simulink model "project"  (R2020a)
settings: Solver=ode15s  StartTime=0.0  StopTime=0.1  RelTol=1e-3
settings Model: Creator=M VEMAN SAI PRABHATH  LastModifiedBy=M VEMAN SAI PRABHATH
settings SolverCC: ZeroCrossAlgorithm=Adaptive
settings DebuggingCC: IgnoredZcDiagnostic=none
settings SFSimCC: CustomCodeUndefinedFunction=UseInterfaceOnly

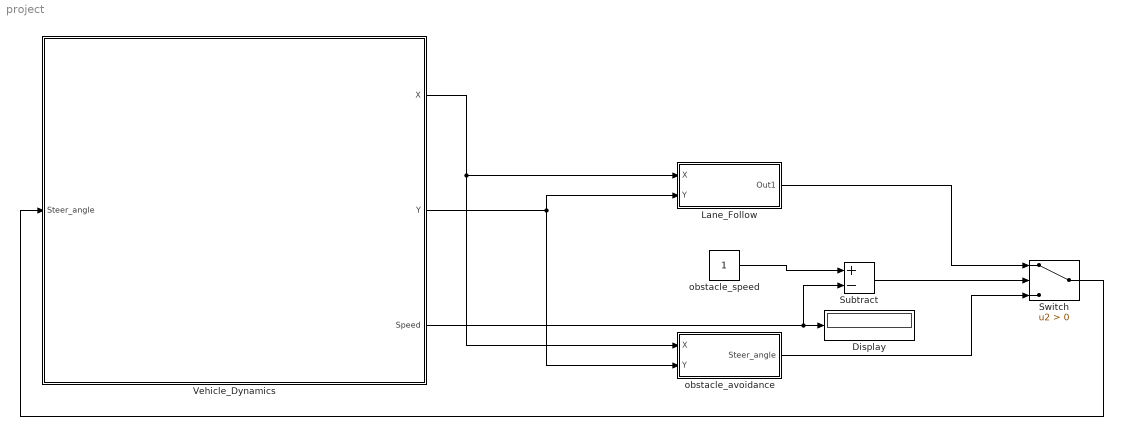
== system project ==
  Display : Display
  Lane_Follow : Subsystem
  Subtract : Sum  Inputs=+-
  Switch : Switch  Criteria=u2 > Threshold
  Vehicle_Dynamics : Subsystem
  obstacle_avoidance : Subsystem
  obstacle_speed : Constant
  wires:
  Vehicle_Dynamics/1(X) -> obstacle_avoidance/1(X), Lane_Follow/1(X)
  Vehicle_Dynamics/2(Y) -> obstacle_avoidance/2(Y), Lane_Follow/2(Y)
  Vehicle_Dynamics/3(Speed) -> Subtract/2, Display/1
  obstacle_speed/1 -> Subtract/1
  Subtract/1 -> Switch/2
  Switch/1 -> Vehicle_Dynamics/1(Steer_angle)
  Lane_Follow/1(Out1) -> Switch/1
  obstacle_avoidance/1(Steer_angle) -> Switch/3

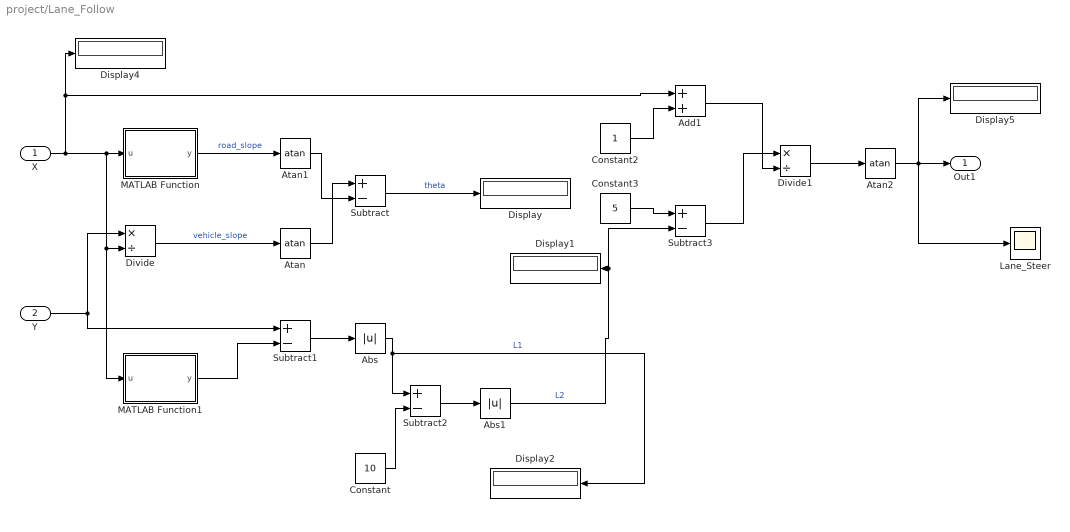
== system project/Lane_Follow ==
  X : Inport
  Y : Inport  Port=2
  Abs : Abs
  Abs1 : Abs
  Add1 : Sum
  Atan : Trigonometry  Operator=atan
  Atan1 : Trigonometry  Operator=atan
  Atan2 : Trigonometry  Operator=atan
  Constant : Constant  Value=10
  Constant2 : Constant
  Constant3 : Constant  Value=5
  Display{,1..2,4..5} (5 alike) : Display
  Divide : Product  Inputs=*/
  Divide1 : Product  Inputs=*/
  Lane_Steer : Scope
  MATLAB Function : MATLAB Function  TreatAsAtomicUnit=on
  MATLAB Function1 : MATLAB Function  TreatAsAtomicUnit=on
  Subtract{,1..3} (4 alike) : Sum  Inputs=+-
  Out1 : Outport
  wires:
  Y/1 -> Divide/1, Subtract1/1
  X/1 -> Add1/1, Display4/1, MATLAB Function/1(u), MATLAB Function1/1(u), Divide/2
  Divide/1 -> Atan/1  "vehicle_slope"
  MATLAB Function/1(y) -> Atan1/1  "road_slope"
  Atan/1 -> Subtract/1
  Atan1/1 -> Subtract/2
  Subtract/1 -> Display/1  "theta"
  MATLAB Function1/1(y) -> Subtract1/2
  Subtract1/1 -> Abs/1
  Abs/1 -> Display2/1, Subtract2/1  "L1"
  Constant/1 -> Subtract2/2
  Subtract2/1 -> Abs1/1
  Abs1/1 -> Subtract3/2, Display1/1  "L2"
  Constant2/1 -> Add1/2
  Constant3/1 -> Subtract3/1
  Subtract3/1 -> Divide1/1
  Add1/1 -> Divide1/2
  Divide1/1 -> Atan2/1
  Atan2/1 -> Lane_Steer/1, Display5/1, Out1/1

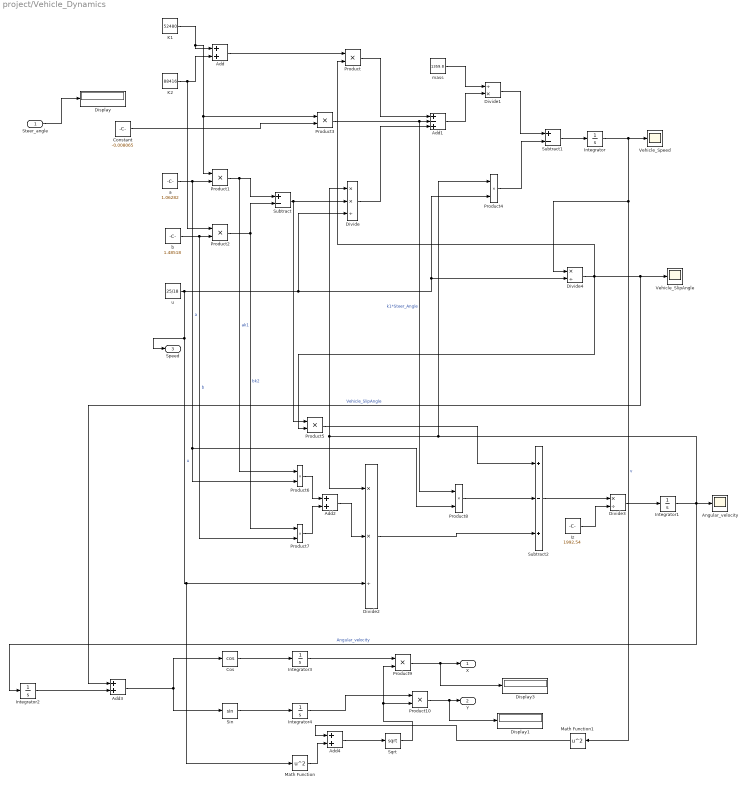
== system project/Vehicle_Dynamics ==
  Steer_angle : Inport
  Add{,2..4} (4 alike) : Sum
  Add1 : Sum  Inputs=+-+
  Angular_velocity : Scope
  Constant : Constant  Value=-0.008065
  Cos : Trigonometry  Operator=cos
  Display : Display
  Display1 : Display
  Display3 : Display
  Divide : Product  Inputs=**/
  Divide1 : Product  Inputs=/*
  Divide2 : Product  Inputs=**/
  Divide3 : Product  Inputs=*/
  Divide4 : Product  Inputs=*/
  Integrator : Integrator  ZeroCross=off
  Integrator{1..4} (4 alike) : Integrator
  Iz : Constant  Value=1992.54
  K1 : Constant  Value=52480
  K2 : Constant  Value=88416
  Math Function : Math  Operator=square  SignedPower=on  SaturateOnIntegerOverflow=on
  Math Function1 : Math  Operator=square  SignedPower=on  SaturateOnIntegerOverflow=on
  Product{,1..10} (11 alike) : Product
  Sin : Trigonometry
  Sqrt : Sqrt  SaturateOnIntegerOverflow=on
  Subtract : Sum  Inputs=+-
  Subtract1 : Sum  Inputs=+-
  Subtract2 : Sum  Inputs=+-+
  Vehicle_SlipAngle : Scope
  Vehicle_Speed : Scope
  a : Constant  Value=1.06282
  b : Constant  Value=1.48518
  mass : Constant  Value=1359.8
  u : Constant  Value=25/18
  X : Outport  VectorParamsAs1DForOutWhenUnconnected=off
  Y : Outport  Port=2  VectorParamsAs1DForOutWhenUnconnected=off
  Speed : Outport  Port=3
  wires:
  u/1 -> Speed/1, Math Function/1, Divide2/3, Divide4/2, Product4/2, Divide/3  "u"
  mass/1 -> Divide1/1
  Subtract/1 -> Product5/1, Divide/2
  Add/1 -> Product/1
  K2/1 -> Product2/1, Add/2
  Product2/1 -> Product7/1, Subtract/2  "bk2"
  K1/1 -> Product3/1, Product1/1, Add/1
  b/1 -> Product7/2, Product2/2  "b"
  Product1/1 -> Product6/1, Subtract/1  "ak1"
  Add1/1 -> Divide1/2
  Divide4/1 -> Product5/2, Add3/1, Vehicle_SlipAngle/1, Product/2  "Vehicle_SlipAngle"
  Subtract1/1 -> Integrator/1
  Divide1/1 -> Subtract1/1
  Product4/1 -> Subtract1/2
  Divide/1 -> Add1/3
  Product/1 -> Add1/1
  Product3/1 -> Product8/1, Add1/2  "k1*Steer_Angle"
  a/1 -> Product8/2, Product6/2, Product1/2  "a"
  Product6/1 -> Add2/1
  Product7/1 -> Add2/2
  Add2/1 -> Divide2/2
  Integrator1/1 -> Integrator2/1, Product4/1, Divide2/1, Divide/1, Angular_velocity/1  "Angular_velocity"
  Divide2/1 -> Subtract2/3
  Product5/1 -> Subtract2/1
  Product8/1 -> Subtract2/2
  Subtract2/1 -> Divide3/1
  Iz/1 -> Divide3/2
  Divide3/1 -> Integrator1/1
  Integrator/1 -> Math Function1/1, Divide4/1, Vehicle_Speed/1  "v"
  Integrator2/1 -> Add3/2
  Add3/1 -> Sin/1, Cos/1
  Cos/1 -> Integrator3/1
  Sin/1 -> Integrator4/1
  Math Function1/1 -> Add4/1
  Math Function/1 -> Add4/2
  Add4/1 -> Sqrt/1
  Sqrt/1 -> Product10/2, Product9/2
  Integrator3/1 -> Product9/1
  Integrator4/1 -> Product10/1
  Product9/1 -> Display3/1, X/1
  Product10/1 -> Display1/1, Y/1
  Constant/1 -> Product3/2
  Steer_angle/1 -> Display/1

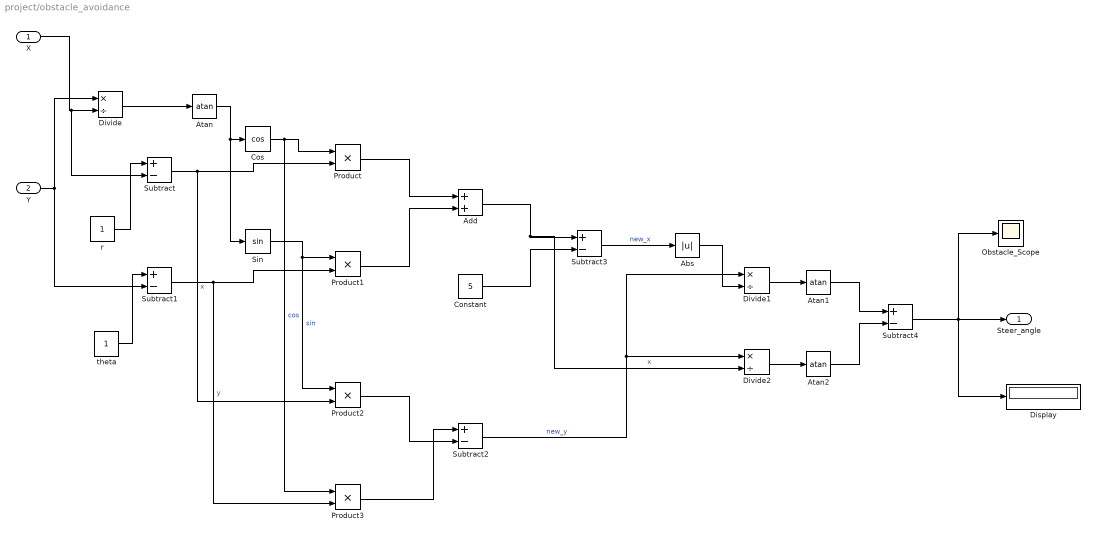
== system project/obstacle_avoidance ==
  X : Inport
  Y : Inport  Port=2
  Abs : Abs
  Add : Sum
  Atan : Trigonometry  Operator=atan
  Atan1 : Trigonometry  Operator=atan
  Atan2 : Trigonometry  Operator=atan
  Constant : Constant  Value=5
  Cos : Trigonometry  Operator=cos
  Display : Display
  Divide : Product  Inputs=*/
  Divide1 : Product  Inputs=*/
  Divide2 : Product  Inputs=*/
  Obstacle_Scope : Scope
  Product{,1..3} (4 alike) : Product
  Sin : Trigonometry
  Subtract{,1..4} (5 alike) : Sum  Inputs=+-
  r : Constant
  theta : Constant
  Steer_angle : Outport  VectorParamsAs1DForOutWhenUnconnected=off
  wires:
  X/1 -> Subtract/2, Divide/2
  Y/1 -> Subtract1/2, Divide/1
  Divide/1 -> Atan/1
  r/1 -> Subtract/1
  Atan/1 -> Sin/1, Cos/1
  Cos/1 -> Product3/1, Product/1  "cos"
  Subtract/1 -> Product2/2, Product/2  "x"
  theta/1 -> Subtract1/1
  Subtract1/1 -> Product3/2, Product1/2  "y"
  Sin/1 -> Product2/1, Product1/1  "sin"
  Product/1 -> Add/1
  Product1/1 -> Add/2
  Product2/1 -> Subtract2/2
  Product3/1 -> Subtract2/1
  Constant/1 -> Subtract3/2
  Add/1 -> Divide2/2, Subtract3/1  "x"
  Subtract3/1 -> Abs/1  "new_x"
  Abs/1 -> Divide1/2
  Subtract2/1 -> Divide1/1, Divide2/1  "new_y"
  Divide1/1 -> Atan1/1
  Divide2/1 -> Atan2/1
  Atan1/1 -> Subtract4/1
  Atan2/1 -> Subtract4/2
  Subtract4/1 -> Obstacle_Scope/1, Display/1, Steer_angle/1

== matlab function project/Lane_Follow/MATLAB Function ==
  data: u input; y output
function y = fcn(u)

y = (2*u) - 5;

== matlab function project/Lane_Follow/MATLAB Function1 ==
  data: u input; y output
function y = fcn(u)

y = (u*u) - (5*u) + 6;
